simulink model "dcmotor_sim"  (R2020b)
settings: Solver=VariableStepAuto  StartTime=0.0  StopTime=10.0  RelTol=1e-3
values from neighbouring files (symbols this model uses):
  K = 0.05    [sig_gen.m]
undefined symbols (not defined in the file or in its folder): b, J, L
settings Model: Creator=shrin  LastModifiedBy=shrin

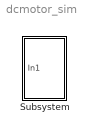
== system dcmotor_sim ==
  Subsystem : Subsystem

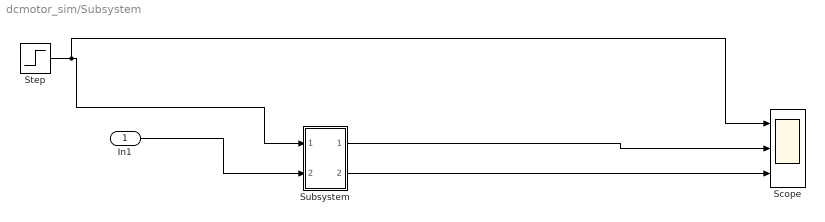
== system dcmotor_sim/Subsystem ==
  In1 : Inport
  Scope : Scope  NumInputPorts=3
  Step : Step  SampleTime=0
  Subsystem : Subsystem
  wires:
  Step/1 -> Subsystem/1(In1), Scope/1
  In1/1 -> Subsystem/2(In2)
  Subsystem/1(Out1) -> Scope/2
  Subsystem/2(Out2) -> Scope/3

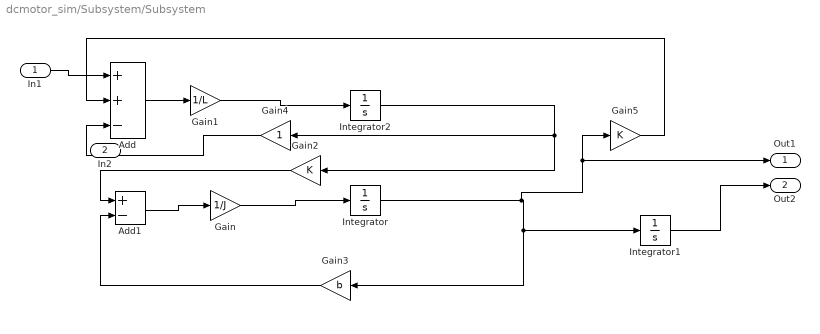
== system dcmotor_sim/Subsystem/Subsystem ==
  In1 : Inport
  In2 : Inport  Port=2
  Add : Sum  Inputs=++-
  Add1 : Sum  Inputs=+-
  Gain : Gain  Gain=1/J
  Gain1 : Gain  Gain=1/L
  Gain2 : Gain  Gain=K
  Gain3 : Gain  Gain=b
  Gain4 : Gain
  Gain5 : Gain  Gain=K
  Integrator : Integrator
  Integrator1 : Integrator
  Integrator2 : Integrator
  Out1 : Outport
  Out2 : Outport  Port=2
  wires:
  Gain3/1 -> Add1/2
  Gain2/1 -> Add1/1
  Gain4/1 -> Add/3
  Integrator2/1 -> Gain4/1, Gain2/1
  Gain/1 -> Integrator/1
  Integrator/1 -> Integrator1/1, Gain3/1, Out1/1, Gain5/1
  Add/1 -> Gain1/1
  Gain1/1 -> Integrator2/1
  Gain5/1 -> Add/2
  Add1/1 -> Gain/1
  In1/1 -> Add/1
  Integrator1/1 -> Out2/1
